simulink model "nonlin_maglev"  (R2025a)
settings: Solver=VariableStepAuto  StartTime=0.0  StopTime=1  RelTol=1e-3
values from neighbouring files (symbols this model uses):
  den = [1 100]    [simulate.m]
  k = 2.9626e-4    (= 0.00029626)    [rhs.m]    (also in simulate.m = -162.15)
  num = [1 30]    [simulate.m]
  us = 0.8475    [simulate.m]
  xs = [0.025;0;0.25;]    [simulate.m]
settings Model: Creator=quintenpienaar  LastModifiedBy=quintenpienaar
settings DataIOCC: SaveOutput=off  SignalLogging=off  DSMLogging=off  SaveTime=off  ReturnWorkspaceOutputs=off

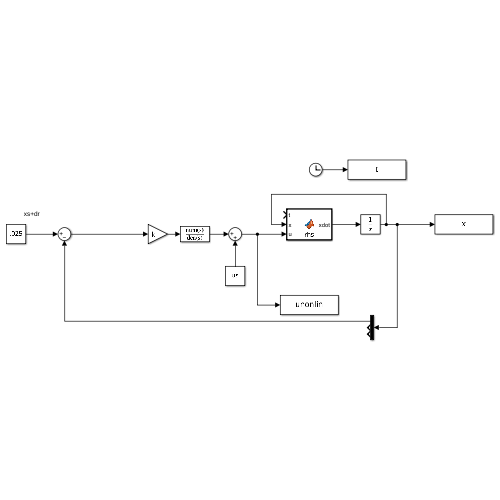
[thumbnail: Simulink's stored preview of the top-level diagram]
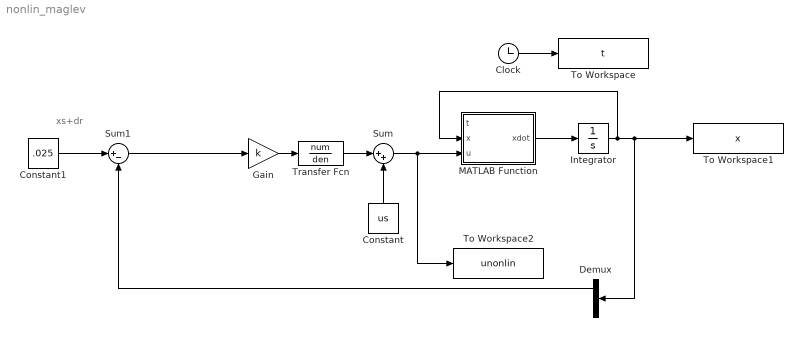
== system nonlin_maglev ==
  note: xs+dr
  Clock : Clock
  Constant : Constant  Value=us
  Constant1 : Constant  Value=.025
  Demux : Demux  Outputs=3
  Gain : Gain  Gain=k
  Integrator : Integrator  InitialCondition=xs - [.001;0;0]
  MATLAB Function : MATLAB Function  TreatAsAtomicUnit=on
  Sum : Sum  Inputs=|++
  Sum1 : Sum  Inputs=|+-
  To Workspace : ToWorkspace  VariableName=t  SampleTime=-1
      settings: Save2DSignal=2-D array (concatenate along first dimension)
  To Workspace1 : ToWorkspace  VariableName=x  SampleTime=-1
      settings: Save2DSignal=2-D array (concatenate along first dimension)
  To Workspace2 : ToWorkspace  VariableName=unonlin  SampleTime=-1
      settings: Save2DSignal=2-D array (concatenate along first dimension)
  Transfer Fcn : TransferFcn  Numerator=num  Denominator=den
  wires:
  MATLAB Function/1(xdot) -> Integrator/1
  Integrator/1 -> MATLAB Function/2(x), Demux/1, To Workspace1/1
  Sum/1 -> To Workspace2/1, MATLAB Function/3(u)
  Constant/1 -> Sum/2
  Clock/1 -> To Workspace/1
  Transfer Fcn/1 -> Sum/1
  Constant1/1 -> Sum1/1
  Gain/1 -> Transfer Fcn/1
  Sum1/1 -> Gain/1
  Demux/1 -> Sum1/2

== matlab function nonlin_maglev/MATLAB Function ==
  data: t input; x input; u input; xdot output
function xdot = rhs(t, x, u)
m = 0.00302; % mass of magnet
g = 9.81;
R = 3.39; % resistance of coil
L = 0.015; %inductance of the coil
k = 2.9626e-4;

xdot = zeros(3, 1);
xdot(1) = x(2);
xdot(2) = (1/m)*((m*g)-(k*((x(3)^2)/x(1)^2)));
xdot(3) = (1/L)*(u - R*x(3));
end
